simulink model "x_lotka_volterra"  (Simulink 7.5)
settings: Solver=ode4  StartTime=0.0  StopTime=200.0  FixedStep=0.05  RelTol=1e-3
PreLoadFcn:
  | alfa=1;beta=-1;gama=-1;delt=1;
libraries: simulink x1
settings Model: Creator=huiliang  LastModifiedBy=huiliang

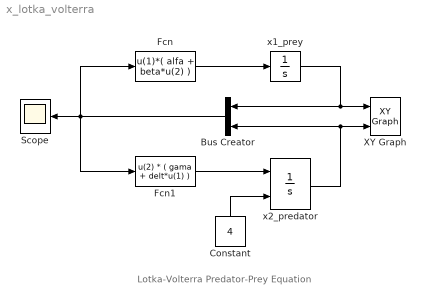
== system x_lotka_volterra ==
  note: Lotka-Volterra Predator-Prey Equation
  Bus Creator : BusCreator  Inputs=2
  Constant : Constant  Value=4  OutDataType=fixdt(1, 16)  OutScaling=2^0
  Fcn : Fcn  Expr=u(1)*( alfa + beta*u(2) )
  Fcn1 : Fcn  Expr=u(2) * ( gama + delt*u(1) )
  Scope : Scope
      settings: YMin=-0.1  YMax=8
  XY Graph : simulink/Sinks/XY Graph  SystemSampleTime=-1  xmin=-0.05  xmax=8  ymin=-0.05  ymax=8  st=-1
  x1_prey : Integrator  InitialCondition=1.5
  x2_predator : Integrator  InitialConditionSource=external  InitialCondition=1
  wires:
  x1_prey/1 -> Bus Creator/1, XY Graph/1
  x2_predator/1 -> Bus Creator/2, XY Graph/2
  Fcn/1 -> x1_prey/1
  Fcn1/1 -> x2_predator/1
  Bus Creator/1 -> Fcn/1, Fcn1/1, Scope/1
  Constant/1 -> x2_predator/2
